simulink model "wen_2016_TPEL_No1"  (R2016b)
settings: Solver=ode4  StartTime=0.0  StopTime=2  FixedStep=Ts  RelTol=1e-3
values from neighbouring files (symbols this model uses):
  deg_per_A = 0+90    (= 90)    [wen_2016_TPEL_No1_m.m]
  deg_per_B = +120+90    (= 210)    [wen_2016_TPEL_No1_m.m]
  deg_per_C = -120+90    (= -30)    [wen_2016_TPEL_No1_m.m]
  f_per = f_dq_i - f0    [wen_2016_TPEL_No1_m.m]
  idref = -sqrt(2) * Ib    [wen_2016_TPEL_No1_m.m]    (also in xin_2017_CSEE_No5_m.m = sqrt(2) * Ib; xin_2017_m.m = sqrt(2) * Ib)
  iqref = 0    [wen_2016_TPEL_No1_m.m]    (also in xin_2017_CSEE_No5_m.m; xin_2017_m.m)
  Ki = 15    [wen_2016_TPEL_No1_m.m]
  Ki_PLL = 991    [wen_2016_TPEL_No1_m.m]    (also in xin_2017_CSEE_No5_m.m = 3020; xin_2017_m.m = 3020)
  Ki_PLL_m = 0.001    [wen_2016_TPEL_No1_m.m]
  Kp = 0.6    [wen_2016_TPEL_No1_m.m]
  Kp_PLL = 4.46    [wen_2016_TPEL_No1_m.m]    (also in xin_2017_CSEE_No5_m.m = 2.5; xin_2017_m.m = 2.5)
  Kp_PLL_m = 0.001    [wen_2016_TPEL_No1_m.m]
  L = 0.1 * Lb    (= 0.000303094673624)    [wen_2016_TPEL_No1_m.m]
  Lf = 0.2 * Lb    (= 0.000606189347248)    [xin_2017_CSEE_No5_m.m]    (also in xin_2017_m.m)
  omega_0 = 2*pi*50    (= 314.159265359)    [wen_2016_TPEL_No1_m.m]    (also in xin_2017_CSEE_No5_m.m; xin_2017_m.m)
  Ts = 1e-4    (= 0.0001)    [wen_2016_TPEL_No1_m.m]    (also in xin_2017_CSEE_No5_m.m; xin_2017_m.m = 5e-06)
  U_per = Us*0.01    [wen_2016_TPEL_No1_m.m]
  Udc = 800    [wen_2016_TPEL_No1_m.m]    (also in xin_2017_CSEE_No5_m.m = 1; xin_2017_m.m = 1000)
  Us = 690/sqrt(3)*sqrt(2)    [wen_2016_TPEL_No1_m.m]    (also in xin_2017_CSEE_No5_m.m; xin_2017_m.m)
libraries: powerlib x15, powerlib_meascontrol x1, powerlib_extras x1
Description:
  | Copyright 2008-2015 The MathWorks, Inc.
settings Model: ExtModeTrigMode=oneshot  ExtModeArmWhenConnect=off  ExtModeAutoUpdateStatusClock=off  Creator=MathWorks  LastModifiedBy=tommy
settings DataIOCC: SaveFinalState=on  SaveFormat=StructureWithTime  SignalLoggingSaveFormat=ModelDataLogs  SignalLogging=off  DSMLogging=off  SaveTime=off  SignalLoggingName=sigsOut
settings OptimizationCC: BlockReduction=off  BooleanDataType=off  ExpressionDepthLimit=2147483647  InitFltsAndDblsToZero=on  EfficientMapNaN2IntZero=off  LifeSpan=inf
settings DebuggingCC: SaveWithParameterizedLinksMsg=none  UnderspecifiedInitializationDetection=Classic  MergeDetectMultiDrivingBlocksExec=none  CheckExecutionContextPreStartOutputMsg=on  CheckExecutionContextRuntimeOutputMsg=on  SignalResolutionControl=TryResolveAllWithWarning  MultiTaskDSMMsg=warning  MultiTaskCondExecSysMsg=none  FcnCallInpInsideContextMsg=warning  AllowSymbolicDim=off  StateNameClashWarn=warning  SFUnexpectedBacktrackingDiag=warning  SFNoUnconditionalDefaultTransitionDiag=warning  SFExecutionAtInitializationDiag=none
settings HardwareCC: ProdBitPerPointer=32  ProdBitPerSizeT=32  ProdBitPerPtrDiffT=32  ProdLargestAtomicFloat=None  ProdIntDivRoundTo=Undefined  ProdEndianess=Unspecified  ProdWordSize=32  ProdHWDeviceType=32-bit Generic  TargetUnknown=on
settings ModelReferenceCC: PropagateSignalLabelsOutOfModel=off
settings GRTTargetCC: TargetFcnLib=ansi_tfl_tmw.mat  TargetLangStandard=C89/C90 (ANSI)  GeneratePreprocessorConditionals=Disable all  CombineOutputUpdateFcns=off  GRTInterface=on
settings ConfigComp: CovMetricSettings=dw  CovHtmlReporting=on  CovSaveCumulativeToWorkspaceVar=on  CovSaveSingleToWorkspaceVar=on  CovExternalEMLEnable=off  CovSFcnEnable=off

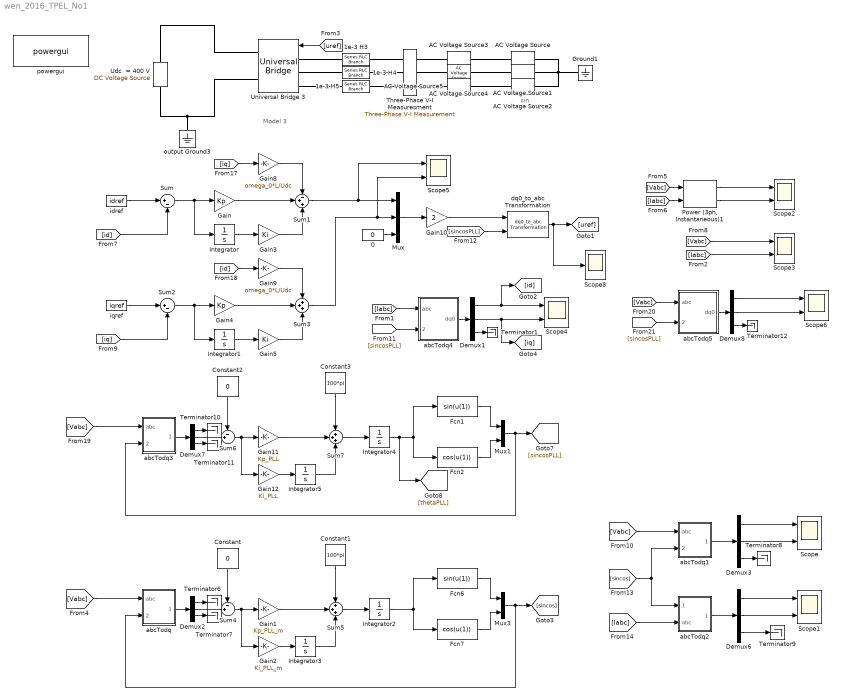
== system wen_2016_TPEL_No1 ==
  note: sin
  note: Model 3
  0 : Constant  Value=0
  1e-3 H3 : powerlib/Elements/Series RLC Branch  LConnTagsString=__new0  RConnTagsString=__new0  BranchType=L  Resistance=1e-3  Inductance=L  SetiL0=off  InitialCurrent=0  Capacitance=1e-6  Setx0=off  InitialVoltage=0  Measurements=None
  1e-3 H4 : powerlib/Elements/Series RLC Branch  LConnTagsString=__new0  RConnTagsString=__new0  BranchType=L  Resistance=Lf  Inductance=L  SetiL0=off  InitialCurrent=0  Capacitance=1e-6  Setx0=off  InitialVoltage=0  Measurements=None
  1e-3 H5 : powerlib/Elements/Series RLC Branch  LConnTagsString=__new0  RConnTagsString=__new0  BranchType=L  Resistance=1e-3  Inductance=L  SetiL0=off  InitialCurrent=0  Capacitance=1e-6  Setx0=off  InitialVoltage=0  Measurements=None
  AC Voltage Source : powerlib/Electrical Sources/AC Voltage Source  Amplitude=Us  Phase=0  Frequency=50  SampleTime=Ts  Measurements=None  BusType=swing  Pref=10e3  Qref=0  Qmin=-inf  Qmax=+inf
  AC Voltage Source1 : powerlib/Electrical Sources/AC Voltage Source  Amplitude=Us  Phase=-120  Frequency=50  SampleTime=Ts  Measurements=None  BusType=swing  Pref=10e3  Qref=0  Qmin=-inf  Qmax=+inf
  AC Voltage Source2 : powerlib/Electrical Sources/AC Voltage Source  Amplitude=Us  Phase=120  Frequency=50  SampleTime=Ts  Measurements=None  BusType=swing  Pref=10e3  Qref=0  Qmin=-inf  Qmax=+inf
  AC Voltage Source3 : powerlib/Electrical Sources/AC Voltage Source  Amplitude=U_per  Phase=deg_per_A  Frequency=f_per  SampleTime=Ts  Measurements=None  BusType=swing  Pref=10e3  Qref=0  Qmin=-inf  Qmax=+inf
  AC Voltage Source4 : powerlib/Electrical Sources/AC Voltage Source  Amplitude=U_per  Phase=deg_per_B  Frequency=f_per  SampleTime=Ts  Measurements=None  BusType=swing  Pref=10e3  Qref=0  Qmin=-inf  Qmax=+inf
  AC Voltage Source5 : powerlib/Electrical Sources/AC Voltage Source  Amplitude=U_per  Phase=deg_per_C  Frequency=f_per  SampleTime=Ts  Measurements=None  BusType=swing  Pref=10e3  Qref=0  Qmin=-inf  Qmax=+inf
  Constant : Constant  Value=0
  Constant1 : Constant  Value=100*pi
  Constant2 : Constant  Value=0
  Constant3 : Constant  Value=100*pi
  Demux{1..3,6..8} (6 alike) : Demux  Outputs=3
  Fcn1 : Fcn  Expr=sin(u(1))
  Fcn2 : Fcn  Expr=cos(u(1))
  Fcn6 : Fcn  Expr=sin(u(1))
  Fcn7 : Fcn  Expr=cos(u(1))
  Gain : Gain  Gain=Kp
  Gain1 : Gain  Gain=Kp_PLL_m
  Gain10 : Gain  Gain=2
  Gain11 : Gain  Gain=Kp_PLL
  Gain12 : Gain  Gain=Ki_PLL
  Gain2 : Gain  Gain=Ki_PLL_m
  Gain3 : Gain  Gain=Ki
  Gain4 : Gain  Gain=Kp
  Gain5 : Gain  Gain=Ki
  Gain8 : Gain  Gain=omega_0*L/Udc
  Gain9 : Gain  Gain=omega_0*L/Udc
  Ground1 : powerlib/Elements/Ground  LConnTagsString=a
  Integrator : Integrator  UpperSaturationLimit=50  LowerSaturationLimit=-50
  Integrator1 : Integrator  UpperSaturationLimit=50  LowerSaturationLimit=-50
  Integrator{2..5} (4 alike) : Integrator
  Mux : Mux  Inputs=3
  Mux1 : Mux  Inputs=2
  Mux3 : Mux  Inputs=2
  "Power (3ph, Instantaneous)1" : powerlib_meascontrol/Measurements/Power (3ph, Instantaneous)
  Scope{,1..6} (7 alike) : Scope  NumInputPorts=2
  Scope8 : Scope
  Sum : Sum  Inputs=|+-
  Sum1 : Sum  Inputs=-++
  Sum2 : Sum  Inputs=|+-
  Sum3 : Sum  Inputs=+++
  Sum4 : Sum  Inputs=-+|
  Sum5 : Sum  Inputs=+++
  Sum6 : Sum  Inputs=-+|
  Sum7 : Sum  Inputs=+++
  Terminator{1,6..12} (8 alike) : Terminator
  Three-Phase V-I Measuresment : powerlib/Measurements/Three-Phase V-I Measurement  VoltageMeasurement=phase-to-ground  SetLabelV=on  LabelV=Vabc  Vpu=off  VpuLL=off  CurrentMeasurement=yes  SetLabelI=on  LabelI=Iabc  Ipu=off  Pbase=100e6  Vbase=500e3  OutputType=Complex  PhasorSimulation=off  PSBequivalent=0
  Udc  = 400 V : powerlib/Electrical Sources/DC Voltage Source  Description=source block  Amplitude=Udc  Measurements=None
      settings: AttributesFormatString=\n
  Universal Bridge 3 : powerlib/Power Electronics/Universal Bridge  Arms=3  SnubberResistance=10000  SnubberCapacitance=inf  Device=Average-model based VSC  Ron=1e-4  Lon=0  ForwardVoltages="[  1  1  ]"  ForwardVoltage=.8  GTOparameters=[ 10e-6 , 20e-6 ]  IGBTparameters=[ 1e-6 , 2e-6 ]  Measurements=None  Measurements_2=None  converterType=Rectifier
      settings: AttributesFormatString=Device: %<Device>
  abcTodq : Subsystem
  abcTodq1 : Subsystem
  abcTodq2 : Subsystem
  abcTodq3 : Subsystem
  abcTodq4 : Subsystem
  abcTodq5 : Subsystem
  dq0_to_abc Transformation : powerlib_extras/Measurements/dq0_to_abc Transformation
  idref : Constant  Value=idref
  "iqref " : Constant  Value=iqref
  output Ground3 : powerlib/Elements/Ground  LConnTagsString=a
  powergui : powerlib/powergui  Priority=2  SimulationMode=Discrete  SolverType=Tustin  SampleTime=Ts  frequency=60  SPID=off  DisableSnubberDevices=off  DisableRonSwitches=off  DisableVfSwitches=off  SwTol=0  DisplayEquations=off  Interpol=off  ExternalGateDelay=off  methode=off  Ts=0  FunctionMessages=off  echomessages=off  HookPort=off  EnableUseOfTLC=off  x0status=blocks  frequencyindice=50  Pbase=100e6  ErrMax=1e-4  Iterations=50  UnitsV=kV  UnitsW=MW  buscounter=0  RestoreLinks=warning  ResistiveCurrentMeasurement=off  Frange=[0:2:500]  Ylog=off  Xlog=off  ShowGrid=off  save=off  variable=ZData  structure=UI  ZoomFFT=off  StartTime=2  cycles=50  DisplayStyle=2  fundamental=50  FreqAxis=off  MaxFrequency=5000  frequencyindicesteady=1  RmsSteady=1  display=off
  wires:
  [uref] -> Universal Bridge 3/1
  [Iabc] -> abcTodq4/1(abc)
  Demux1/2 -> [iq], Scope4/2
  Demux1/1 -> [id], Scope4/1
  idref/1 -> Sum/1
  Sum/1 -> Gain/1, Integrator/1
  Integrator/1 -> Gain3/1
  "iqref "/1 -> Sum2/1
  Sum2/1 -> Gain4/1, Integrator1/1
  Integrator1/1 -> Gain5/1
  0/1 -> Mux/3
  [sincosPLL] -> dq0_to_abc Transformation/2
  dq0_to_abc Transformation/1 -> Scope8/1, [uref]
  Demux1/3 -> Terminator1/1
  [Vabc] -> Scope3/1
  [Iabc] -> "Power (3ph, Instantaneous)1"/2
  "Power (3ph, Instantaneous)1"/2 -> Scope2/2
  [Vabc] -> "Power (3ph, Instantaneous)1"/1
  "Power (3ph, Instantaneous)1"/1 -> Scope2/1
  [Iabc] -> Scope3/2
  [iq] -> Gain8/1
  Gain8/1 -> Sum1/1
  Gain/1 -> Sum1/2
  Gain3/1 -> Sum1/3
  [id] -> Gain9/1
  Gain9/1 -> Sum3/1
  Gain4/1 -> Sum3/2
  Gain5/1 -> Sum3/3
  Sum3/1 -> Scope5/2, Mux/2
  Sum1/1 -> Scope5/1, Mux/1
  Mux/1 -> Gain10/1
  abcTodq/1(dq0) -> Demux2/1
  Constant/1 -> Sum4/1
  Demux2/2 -> Sum4/2
  Sum4/1 -> Gain2/1, Gain1/1
  Integrator2/1 -> Fcn6/1, Fcn7/1
  Fcn6/1 -> Mux3/1
  Fcn7/1 -> Mux3/2
  Mux3/1 -> [sincos], abcTodq/2(sin_cos)
  Gain1/1 -> Sum5/2
  Sum5/1 -> Integrator2/1
  Constant1/1 -> Sum5/1
  [Vabc] -> abcTodq/1(abc)
  Gain2/1 -> Integrator3/1
  Integrator3/1 -> Sum5/3
  [Vabc] -> abcTodq1/1(abc)
  [sincos] -> abcTodq1/2(sin_cos), abcTodq2/1(sin_cos)
  abcTodq1/1(dq0) -> Demux3/1
  [Iabc] -> abcTodq2/2(abc)
  abcTodq2/1(dq0) -> Demux6/1
  Demux3/1 -> Scope/1
  Demux3/2 -> Scope/2
  Demux3/3 -> Terminator8/1
  Demux6/1 -> Scope1/1
  Demux6/2 -> Scope1/2
  Demux6/3 -> Terminator9/1
  Demux2/1 -> Terminator6/1
  Demux2/3 -> Terminator7/1
  abcTodq3/1(dq0) -> Demux7/1
  Constant2/1 -> Sum6/1
  Demux7/2 -> Sum6/2
  Sum6/1 -> Gain12/1, Gain11/1
  Integrator4/1 -> [thetaPLL], Fcn1/1, Fcn2/1
  Fcn1/1 -> Mux1/1
  Fcn2/1 -> Mux1/2
  Mux1/1 -> [sincosPLL], abcTodq3/2(sin_cos)
  Gain11/1 -> Sum7/2
  Sum7/1 -> Integrator4/1
  Constant3/1 -> Sum7/1
  [Vabc] -> abcTodq3/1(abc)
  Gain12/1 -> Integrator5/1
  Integrator5/1 -> Sum7/3
  Demux7/1 -> Terminator10/1
  Demux7/3 -> Terminator11/1
  [sincosPLL] -> abcTodq4/2(sin_cos)
  abcTodq4/1(dq0) -> Demux1/1
  [Vabc] -> abcTodq5/1(abc)
  Demux8/2 -> Scope6/2
  Demux8/1 -> Scope6/1
  Demux8/3 -> Terminator12/1
  [sincosPLL] -> abcTodq5/2(sin_cos)
  abcTodq5/1(dq0) -> Demux8/1
  Gain10/1 -> dq0_to_abc Transformation/1
  [id] -> Sum/2
  [iq] -> Sum2/2
  connections:
  AC Voltage Source/LConn1 -- AC Voltage Source2/LConn1 -- Ground1/LConn1 -- AC Voltage Source1/LConn1
  Udc  = 400 V/LConn1 -- Universal Bridge 3/RConn2 -- output Ground3/LConn1
  Udc  = 400 V/RConn1 -- Universal Bridge 3/RConn1
  1e-3 H3/LConn1 -- Universal Bridge 3/LConn1
  1e-3 H4/LConn1 -- Universal Bridge 3/LConn2
  1e-3 H5/LConn1 -- Universal Bridge 3/LConn3
  AC Voltage Source3/LConn1 -- AC Voltage Source/RConn1
  AC Voltage Source4/LConn1 -- AC Voltage Source1/RConn1
  AC Voltage Source5/LConn1 -- AC Voltage Source2/RConn1
  Three-Phase V-I Measuresment/LConn1 -- 1e-3 H3/RConn1
  Three-Phase V-I Measuresment/LConn2 -- 1e-3 H4/RConn1
  Three-Phase V-I Measuresment/LConn3 -- 1e-3 H5/RConn1
  AC Voltage Source3/RConn1 -- Three-Phase V-I Measuresment/RConn1
  AC Voltage Source4/RConn1 -- Three-Phase V-I Measuresment/RConn2
  AC Voltage Source5/RConn1 -- Three-Phase V-I Measuresment/RConn3

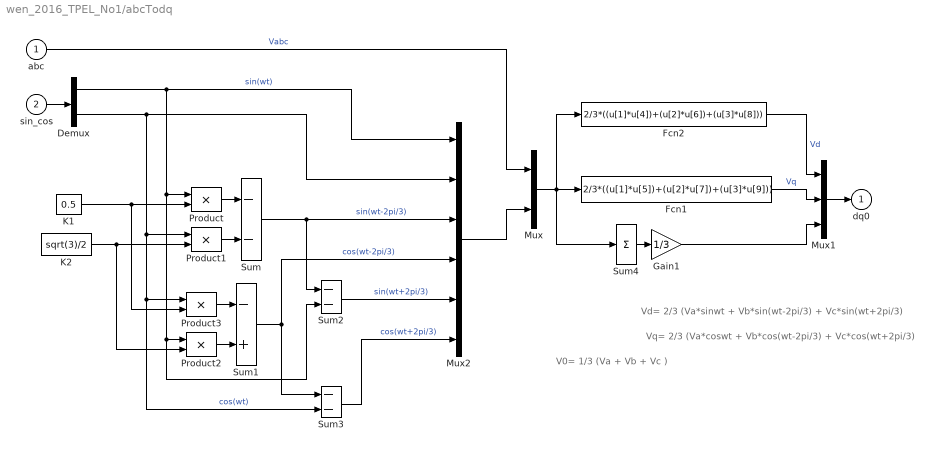
== system wen_2016_TPEL_No1/abcTodq ==
  note: V0= 1/3 (Va + Vb + Vc )
  note: Vd= 2/3 (Va*sinwt + Vb*sin(wt-2pi/3) + Vc*sin(wt+2pi/3)
  note: Vq= 2/3 (Va*coswt + Vb*cos(wt-2pi/3) + Vc*cos(wt+2pi/3)
  abc : Inport  PortDimensions=3
  sin_cos : Inport  Port=2  PortDimensions=2
  Demux : Demux  Outputs=2
  Fcn1 : Fcn  Expr=2/3*((u[1]*u[5])+(u[2]*u[7])+(u[3]*u[9]))
  Fcn2 : Fcn  Expr=2/3*((u[1]*u[4])+(u[2]*u[6])+(u[3]*u[8]))
  Gain1 : Gain  Gain=1/3  SaturateOnIntegerOverflow=on  OutDataTypeStr=Inherit: Same as input  ParamDataTypeStr=Inherit: Same as input
  K1 : Constant  Value=0.5
  K2 : Constant  Value=sqrt(3)/2
  Mux : Mux  Inputs=2
  Mux1 : Mux  Inputs=3
  Mux2 : Mux  Inputs=6
  Product{,1..3} (4 alike) : Product  SaturateOnIntegerOverflow=on  InputSameDT=on  OutDataTypeStr=Inherit: Same as first input
  Sum : Sum  Inputs=--  SaturateOnIntegerOverflow=on  InputSameDT=on  OutDataTypeStr=Inherit: Same as first input
  Sum1 : Sum  Inputs=-+  SaturateOnIntegerOverflow=on  InputSameDT=on  OutDataTypeStr=Inherit: Same as first input
  Sum2 : Sum  Inputs=--  SaturateOnIntegerOverflow=on  InputSameDT=on  OutDataTypeStr=Inherit: Same as first input
  Sum3 : Sum  Inputs=--  SaturateOnIntegerOverflow=on  InputSameDT=on  OutDataTypeStr=Inherit: Same as first input
  Sum4 : Sum  Inputs=1  SaturateOnIntegerOverflow=on  InputSameDT=on  OutDataTypeStr=Inherit: Same as first input
  dq0 : Outport  InitialOutput=0
  wires:
  Gain1/1 -> Mux1/3
  Fcn2/1 -> Mux1/1  "Vd"
  Fcn1/1 -> Mux1/2  "Vq"
  Mux1/1 -> dq0/1
  Sum4/1 -> Gain1/1
  Mux/1 -> Sum4/1, Fcn1/1, Fcn2/1
  Sum1/1 -> Sum3/1, Mux2/4  "cos(wt-2pi/3)"
  Sum/1 -> Sum2/1, Mux2/3  "sin(wt-2pi/3)"
  K2/1 -> Product2/2, Product1/2
  K1/1 -> Product3/2, Product/2
  Sum2/1 -> Mux2/5  "sin(wt+2pi/3)"
  Sum3/1 -> Mux2/6  "cos(wt+2pi/3)"
  Product2/1 -> Sum1/2
  Product3/1 -> Sum1/1
  Product1/1 -> Sum/2
  Product/1 -> Sum/1
  Demux/1 -> Mux2/1, Sum2/2, Product2/1, Product/1  "sin(wt)"
  Demux/2 -> Mux2/2, Product1/1, Product3/1, Sum3/2  "cos(wt)"
  sin_cos/1 -> Demux/1
  Mux2/1 -> Mux/2
  abc/1 -> Mux/1  "Vabc"

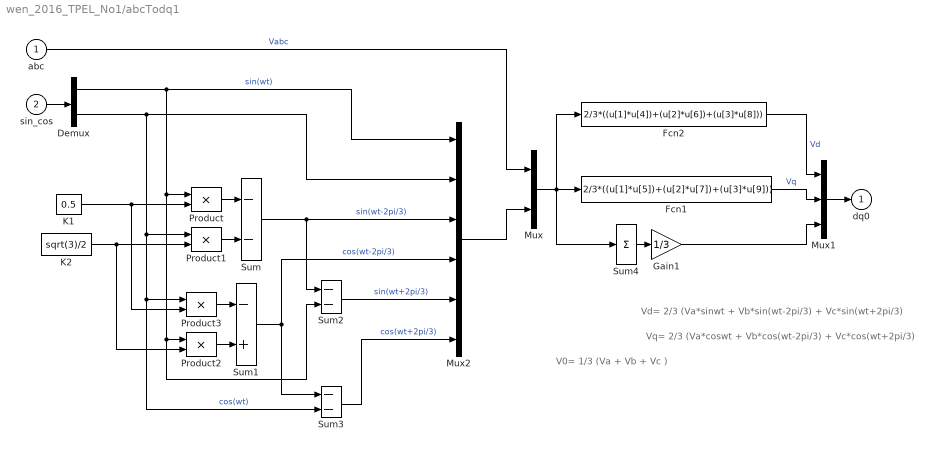
== system wen_2016_TPEL_No1/abcTodq1 ==
  note: V0= 1/3 (Va + Vb + Vc )
  note: Vd= 2/3 (Va*sinwt + Vb*sin(wt-2pi/3) + Vc*sin(wt+2pi/3)
  note: Vq= 2/3 (Va*coswt + Vb*cos(wt-2pi/3) + Vc*cos(wt+2pi/3)
  abc : Inport  PortDimensions=3
  sin_cos : Inport  Port=2  PortDimensions=2
  Demux : Demux  Outputs=2
  Fcn1 : Fcn  Expr=2/3*((u[1]*u[5])+(u[2]*u[7])+(u[3]*u[9]))
  Fcn2 : Fcn  Expr=2/3*((u[1]*u[4])+(u[2]*u[6])+(u[3]*u[8]))
  Gain1 : Gain  Gain=1/3  SaturateOnIntegerOverflow=on  OutDataTypeStr=Inherit: Same as input  ParamDataTypeStr=Inherit: Same as input
  K1 : Constant  Value=0.5
  K2 : Constant  Value=sqrt(3)/2
  Mux : Mux  Inputs=2
  Mux1 : Mux  Inputs=3
  Mux2 : Mux  Inputs=6
  Product{,1..3} (4 alike) : Product  SaturateOnIntegerOverflow=on  InputSameDT=on  OutDataTypeStr=Inherit: Same as first input
  Sum : Sum  Inputs=--  SaturateOnIntegerOverflow=on  InputSameDT=on  OutDataTypeStr=Inherit: Same as first input
  Sum1 : Sum  Inputs=-+  SaturateOnIntegerOverflow=on  InputSameDT=on  OutDataTypeStr=Inherit: Same as first input
  Sum2 : Sum  Inputs=--  SaturateOnIntegerOverflow=on  InputSameDT=on  OutDataTypeStr=Inherit: Same as first input
  Sum3 : Sum  Inputs=--  SaturateOnIntegerOverflow=on  InputSameDT=on  OutDataTypeStr=Inherit: Same as first input
  Sum4 : Sum  Inputs=1  SaturateOnIntegerOverflow=on  InputSameDT=on  OutDataTypeStr=Inherit: Same as first input
  dq0 : Outport  InitialOutput=0
  wires:
  Gain1/1 -> Mux1/3
  Fcn2/1 -> Mux1/1  "Vd"
  Fcn1/1 -> Mux1/2  "Vq"
  Mux1/1 -> dq0/1
  Sum4/1 -> Gain1/1
  Mux/1 -> Sum4/1, Fcn1/1, Fcn2/1
  Sum1/1 -> Sum3/1, Mux2/4  "cos(wt-2pi/3)"
  Sum/1 -> Sum2/1, Mux2/3  "sin(wt-2pi/3)"
  K2/1 -> Product2/2, Product1/2
  K1/1 -> Product3/2, Product/2
  Sum2/1 -> Mux2/5  "sin(wt+2pi/3)"
  Sum3/1 -> Mux2/6  "cos(wt+2pi/3)"
  Product2/1 -> Sum1/2
  Product3/1 -> Sum1/1
  Product1/1 -> Sum/2
  Product/1 -> Sum/1
  Demux/1 -> Mux2/1, Sum2/2, Product2/1, Product/1  "sin(wt)"
  Demux/2 -> Mux2/2, Product1/1, Product3/1, Sum3/2  "cos(wt)"
  sin_cos/1 -> Demux/1
  Mux2/1 -> Mux/2
  abc/1 -> Mux/1  "Vabc"

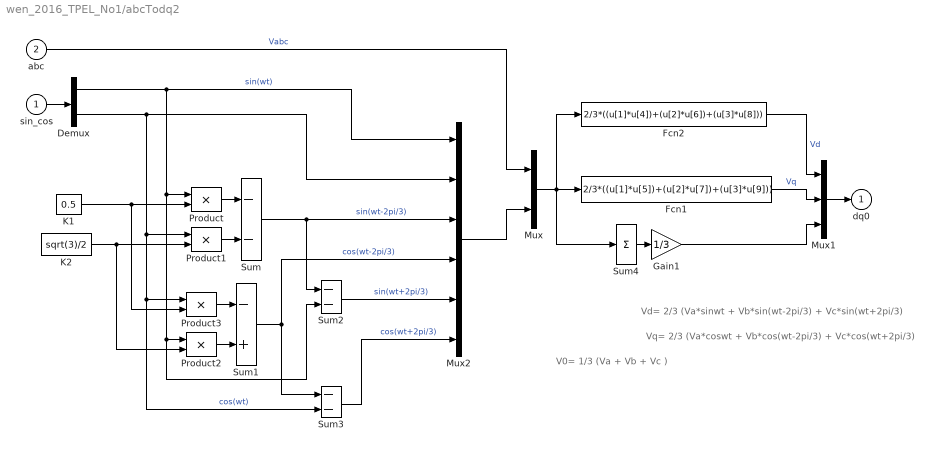
== system wen_2016_TPEL_No1/abcTodq2 ==
  note: V0= 1/3 (Va + Vb + Vc )
  note: Vd= 2/3 (Va*sinwt + Vb*sin(wt-2pi/3) + Vc*sin(wt+2pi/3)
  note: Vq= 2/3 (Va*coswt + Vb*cos(wt-2pi/3) + Vc*cos(wt+2pi/3)
  sin_cos : Inport  PortDimensions=2
  abc : Inport  Port=2  PortDimensions=3
  Demux : Demux  Outputs=2
  Fcn1 : Fcn  Expr=2/3*((u[1]*u[5])+(u[2]*u[7])+(u[3]*u[9]))
  Fcn2 : Fcn  Expr=2/3*((u[1]*u[4])+(u[2]*u[6])+(u[3]*u[8]))
  Gain1 : Gain  Gain=1/3  SaturateOnIntegerOverflow=on  OutDataTypeStr=Inherit: Same as input  ParamDataTypeStr=Inherit: Same as input
  K1 : Constant  Value=0.5
  K2 : Constant  Value=sqrt(3)/2
  Mux : Mux  Inputs=2
  Mux1 : Mux  Inputs=3
  Mux2 : Mux  Inputs=6
  Product{,1..3} (4 alike) : Product  SaturateOnIntegerOverflow=on  InputSameDT=on  OutDataTypeStr=Inherit: Same as first input
  Sum : Sum  Inputs=--  SaturateOnIntegerOverflow=on  InputSameDT=on  OutDataTypeStr=Inherit: Same as first input
  Sum1 : Sum  Inputs=-+  SaturateOnIntegerOverflow=on  InputSameDT=on  OutDataTypeStr=Inherit: Same as first input
  Sum2 : Sum  Inputs=--  SaturateOnIntegerOverflow=on  InputSameDT=on  OutDataTypeStr=Inherit: Same as first input
  Sum3 : Sum  Inputs=--  SaturateOnIntegerOverflow=on  InputSameDT=on  OutDataTypeStr=Inherit: Same as first input
  Sum4 : Sum  Inputs=1  SaturateOnIntegerOverflow=on  InputSameDT=on  OutDataTypeStr=Inherit: Same as first input
  dq0 : Outport  InitialOutput=0
  wires:
  Gain1/1 -> Mux1/3
  Fcn2/1 -> Mux1/1  "Vd"
  Fcn1/1 -> Mux1/2  "Vq"
  Mux1/1 -> dq0/1
  Sum4/1 -> Gain1/1
  Mux/1 -> Sum4/1, Fcn1/1, Fcn2/1
  Sum1/1 -> Sum3/1, Mux2/4  "cos(wt-2pi/3)"
  Sum/1 -> Sum2/1, Mux2/3  "sin(wt-2pi/3)"
  K2/1 -> Product2/2, Product1/2
  K1/1 -> Product3/2, Product/2
  Sum2/1 -> Mux2/5  "sin(wt+2pi/3)"
  Sum3/1 -> Mux2/6  "cos(wt+2pi/3)"
  Product2/1 -> Sum1/2
  Product3/1 -> Sum1/1
  Product1/1 -> Sum/2
  Product/1 -> Sum/1
  Demux/1 -> Mux2/1, Sum2/2, Product2/1, Product/1  "sin(wt)"
  Demux/2 -> Mux2/2, Product1/1, Product3/1, Sum3/2  "cos(wt)"
  sin_cos/1 -> Demux/1
  Mux2/1 -> Mux/2
  abc/1 -> Mux/1  "Vabc"

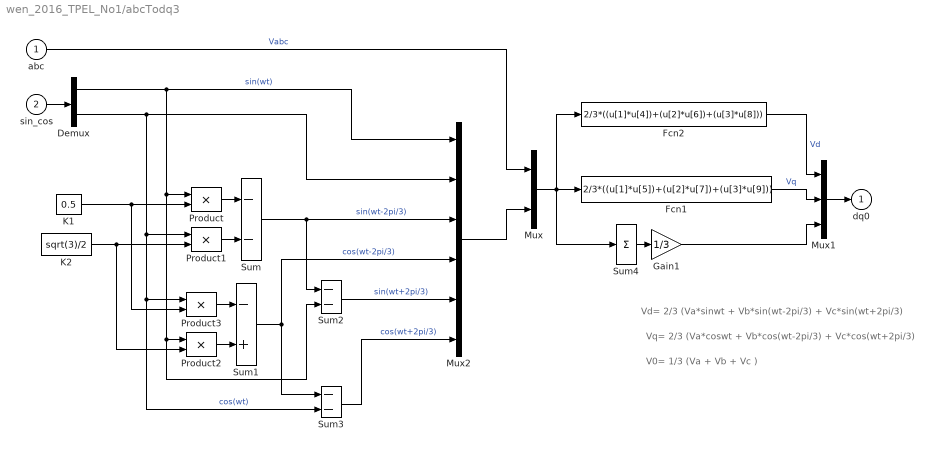
== system wen_2016_TPEL_No1/abcTodq3 ==
  note: V0= 1/3 (Va + Vb + Vc )
  note: Vd= 2/3 (Va*sinwt + Vb*sin(wt-2pi/3) + Vc*sin(wt+2pi/3)
  note: Vq= 2/3 (Va*coswt + Vb*cos(wt-2pi/3) + Vc*cos(wt+2pi/3)
  abc : Inport  PortDimensions=3
  sin_cos : Inport  Port=2  PortDimensions=2
  Demux : Demux  Outputs=2
  Fcn1 : Fcn  Expr=2/3*((u[1]*u[5])+(u[2]*u[7])+(u[3]*u[9]))
  Fcn2 : Fcn  Expr=2/3*((u[1]*u[4])+(u[2]*u[6])+(u[3]*u[8]))
  Gain1 : Gain  Gain=1/3  SaturateOnIntegerOverflow=on  OutDataTypeStr=Inherit: Same as input  ParamDataTypeStr=Inherit: Same as input
  K1 : Constant  Value=0.5
  K2 : Constant  Value=sqrt(3)/2
  Mux : Mux  Inputs=2
  Mux1 : Mux  Inputs=3
  Mux2 : Mux  Inputs=6
  Product{,1..3} (4 alike) : Product  SaturateOnIntegerOverflow=on  InputSameDT=on  OutDataTypeStr=Inherit: Same as first input
  Sum : Sum  Inputs=--  SaturateOnIntegerOverflow=on  InputSameDT=on  OutDataTypeStr=Inherit: Same as first input
  Sum1 : Sum  Inputs=-+  SaturateOnIntegerOverflow=on  InputSameDT=on  OutDataTypeStr=Inherit: Same as first input
  Sum2 : Sum  Inputs=--  SaturateOnIntegerOverflow=on  InputSameDT=on  OutDataTypeStr=Inherit: Same as first input
  Sum3 : Sum  Inputs=--  SaturateOnIntegerOverflow=on  InputSameDT=on  OutDataTypeStr=Inherit: Same as first input
  Sum4 : Sum  Inputs=1  SaturateOnIntegerOverflow=on  InputSameDT=on  OutDataTypeStr=Inherit: Same as first input
  dq0 : Outport  InitialOutput=0
  wires:
  Gain1/1 -> Mux1/3
  Fcn2/1 -> Mux1/1  "Vd"
  Fcn1/1 -> Mux1/2  "Vq"
  Mux1/1 -> dq0/1
  Sum4/1 -> Gain1/1
  Mux/1 -> Sum4/1, Fcn1/1, Fcn2/1
  Sum1/1 -> Sum3/1, Mux2/4  "cos(wt-2pi/3)"
  Sum/1 -> Sum2/1, Mux2/3  "sin(wt-2pi/3)"
  K2/1 -> Product2/2, Product1/2
  K1/1 -> Product3/2, Product/2
  Sum2/1 -> Mux2/5  "sin(wt+2pi/3)"
  Sum3/1 -> Mux2/6  "cos(wt+2pi/3)"
  Product2/1 -> Sum1/2
  Product3/1 -> Sum1/1
  Product1/1 -> Sum/2
  Product/1 -> Sum/1
  Demux/1 -> Mux2/1, Sum2/2, Product2/1, Product/1  "sin(wt)"
  Demux/2 -> Mux2/2, Product1/1, Product3/1, Sum3/2  "cos(wt)"
  sin_cos/1 -> Demux/1
  Mux2/1 -> Mux/2
  abc/1 -> Mux/1  "Vabc"

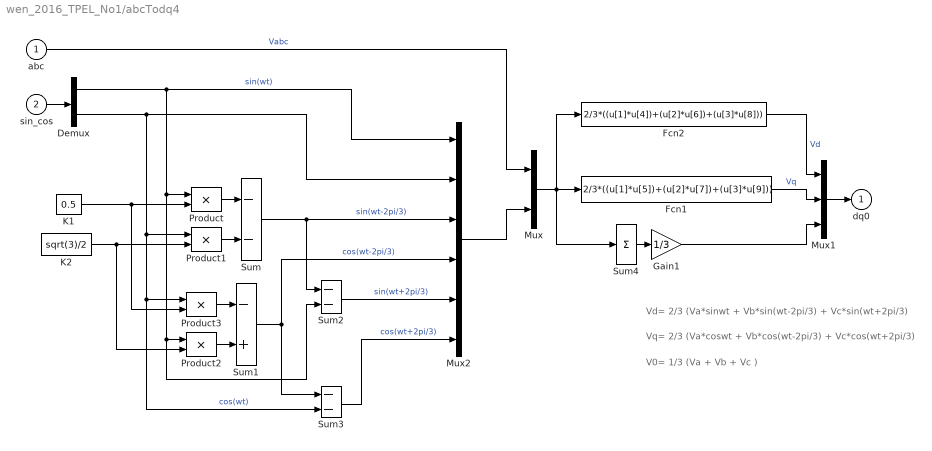
== system wen_2016_TPEL_No1/abcTodq4 ==
  note: V0= 1/3 (Va + Vb + Vc )
  note: Vd= 2/3 (Va*sinwt + Vb*sin(wt-2pi/3) + Vc*sin(wt+2pi/3)
  note: Vq= 2/3 (Va*coswt + Vb*cos(wt-2pi/3) + Vc*cos(wt+2pi/3)
  abc : Inport  PortDimensions=3
  sin_cos : Inport  Port=2  PortDimensions=2
  Demux : Demux  Outputs=2
  Fcn1 : Fcn  Expr=2/3*((u[1]*u[5])+(u[2]*u[7])+(u[3]*u[9]))
  Fcn2 : Fcn  Expr=2/3*((u[1]*u[4])+(u[2]*u[6])+(u[3]*u[8]))
  Gain1 : Gain  Gain=1/3  SaturateOnIntegerOverflow=on  OutDataTypeStr=Inherit: Same as input  ParamDataTypeStr=Inherit: Same as input
  K1 : Constant  Value=0.5
  K2 : Constant  Value=sqrt(3)/2
  Mux : Mux  Inputs=2
  Mux1 : Mux  Inputs=3
  Mux2 : Mux  Inputs=6
  Product{,1..3} (4 alike) : Product  SaturateOnIntegerOverflow=on  InputSameDT=on  OutDataTypeStr=Inherit: Same as first input
  Sum : Sum  Inputs=--  SaturateOnIntegerOverflow=on  InputSameDT=on  OutDataTypeStr=Inherit: Same as first input
  Sum1 : Sum  Inputs=-+  SaturateOnIntegerOverflow=on  InputSameDT=on  OutDataTypeStr=Inherit: Same as first input
  Sum2 : Sum  Inputs=--  SaturateOnIntegerOverflow=on  InputSameDT=on  OutDataTypeStr=Inherit: Same as first input
  Sum3 : Sum  Inputs=--  SaturateOnIntegerOverflow=on  InputSameDT=on  OutDataTypeStr=Inherit: Same as first input
  Sum4 : Sum  Inputs=1  SaturateOnIntegerOverflow=on  InputSameDT=on  OutDataTypeStr=Inherit: Same as first input
  dq0 : Outport  InitialOutput=0
  wires:
  Gain1/1 -> Mux1/3
  Fcn2/1 -> Mux1/1  "Vd"
  Fcn1/1 -> Mux1/2  "Vq"
  Mux1/1 -> dq0/1
  Sum4/1 -> Gain1/1
  Mux/1 -> Sum4/1, Fcn1/1, Fcn2/1
  Sum1/1 -> Sum3/1, Mux2/4  "cos(wt-2pi/3)"
  Sum/1 -> Sum2/1, Mux2/3  "sin(wt-2pi/3)"
  K2/1 -> Product2/2, Product1/2
  K1/1 -> Product3/2, Product/2
  Sum2/1 -> Mux2/5  "sin(wt+2pi/3)"
  Sum3/1 -> Mux2/6  "cos(wt+2pi/3)"
  Product2/1 -> Sum1/2
  Product3/1 -> Sum1/1
  Product1/1 -> Sum/2
  Product/1 -> Sum/1
  Demux/1 -> Mux2/1, Sum2/2, Product2/1, Product/1  "sin(wt)"
  Demux/2 -> Mux2/2, Product1/1, Product3/1, Sum3/2  "cos(wt)"
  sin_cos/1 -> Demux/1
  Mux2/1 -> Mux/2
  abc/1 -> Mux/1  "Vabc"

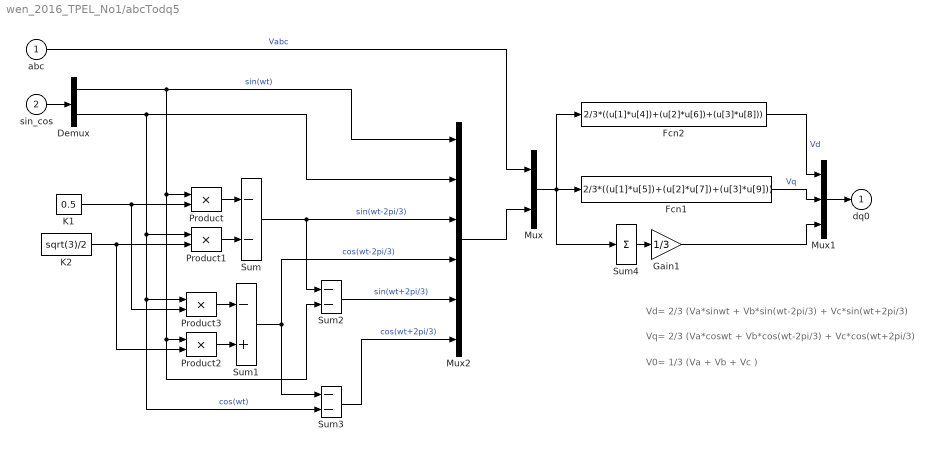
== system wen_2016_TPEL_No1/abcTodq5 ==
  note: V0= 1/3 (Va + Vb + Vc )
  note: Vd= 2/3 (Va*sinwt + Vb*sin(wt-2pi/3) + Vc*sin(wt+2pi/3)
  note: Vq= 2/3 (Va*coswt + Vb*cos(wt-2pi/3) + Vc*cos(wt+2pi/3)
  abc : Inport  PortDimensions=3
  sin_cos : Inport  Port=2  PortDimensions=2
  Demux : Demux  Outputs=2
  Fcn1 : Fcn  Expr=2/3*((u[1]*u[5])+(u[2]*u[7])+(u[3]*u[9]))
  Fcn2 : Fcn  Expr=2/3*((u[1]*u[4])+(u[2]*u[6])+(u[3]*u[8]))
  Gain1 : Gain  Gain=1/3  SaturateOnIntegerOverflow=on  OutDataTypeStr=Inherit: Same as input  ParamDataTypeStr=Inherit: Same as input
  K1 : Constant  Value=0.5
  K2 : Constant  Value=sqrt(3)/2
  Mux : Mux  Inputs=2
  Mux1 : Mux  Inputs=3
  Mux2 : Mux  Inputs=6
  Product{,1..3} (4 alike) : Product  SaturateOnIntegerOverflow=on  InputSameDT=on  OutDataTypeStr=Inherit: Same as first input
  Sum : Sum  Inputs=--  SaturateOnIntegerOverflow=on  InputSameDT=on  OutDataTypeStr=Inherit: Same as first input
  Sum1 : Sum  Inputs=-+  SaturateOnIntegerOverflow=on  InputSameDT=on  OutDataTypeStr=Inherit: Same as first input
  Sum2 : Sum  Inputs=--  SaturateOnIntegerOverflow=on  InputSameDT=on  OutDataTypeStr=Inherit: Same as first input
  Sum3 : Sum  Inputs=--  SaturateOnIntegerOverflow=on  InputSameDT=on  OutDataTypeStr=Inherit: Same as first input
  Sum4 : Sum  Inputs=1  SaturateOnIntegerOverflow=on  InputSameDT=on  OutDataTypeStr=Inherit: Same as first input
  dq0 : Outport  InitialOutput=0
  wires:
  Gain1/1 -> Mux1/3
  Fcn2/1 -> Mux1/1  "Vd"
  Fcn1/1 -> Mux1/2  "Vq"
  Mux1/1 -> dq0/1
  Sum4/1 -> Gain1/1
  Mux/1 -> Sum4/1, Fcn1/1, Fcn2/1
  Sum1/1 -> Sum3/1, Mux2/4  "cos(wt-2pi/3)"
  Sum/1 -> Sum2/1, Mux2/3  "sin(wt-2pi/3)"
  K2/1 -> Product2/2, Product1/2
  K1/1 -> Product3/2, Product/2
  Sum2/1 -> Mux2/5  "sin(wt+2pi/3)"
  Sum3/1 -> Mux2/6  "cos(wt+2pi/3)"
  Product2/1 -> Sum1/2
  Product3/1 -> Sum1/1
  Product1/1 -> Sum/2
  Product/1 -> Sum/1
  Demux/1 -> Mux2/1, Sum2/2, Product2/1, Product/1  "sin(wt)"
  Demux/2 -> Mux2/2, Product1/1, Product3/1, Sum3/2  "cos(wt)"
  sin_cos/1 -> Demux/1
  Mux2/1 -> Mux/2
  abc/1 -> Mux/1  "Vabc"
